simulink model "V1"  (Simulink 8.9)
settings: Solver=VariableStepAuto  StartTime=0.0  StopTime=5  RelTol=1e-3
values from neighbouring files (symbols this model uses):
  Fz = m*g/2    (= 3924)    [variabeln.m]    (also in variabeln_v2.m)
  J = 1    [variabeln.m]    (also in variabeln_v2.m)
  m = 800    [variabeln.m]    (also in variabeln_v2.m)
  r = 0.25    [variabeln.m]    (also in variabeln_v2.m)
  theta1 = 1.28    [variabeln.m]    (also in variabeln_v2.m)
  theta2 = 23.99    [variabeln.m]    (also in variabeln_v2.m)
  theta3 = 0.52    [variabeln.m]    (also in variabeln_v2.m)
  v0 = 10    [variabeln.m]    (also in variabeln_v2.m = 50)
settings Model: Creator=frede  LastModifiedBy=frede
settings DataIOCC: LimitDataPoints=off  SaveFormat=Dataset  SignalLoggingSaveFormat=Dataset
settings OptimizationCC: LifeSpan=auto
settings DebuggingCC: UnderspecifiedInitializationDetection=Simplified  MergeDetectMultiDrivingBlocksExec=error  FcnCallInpInsideContextMsg=error  StateNameClashWarn=none  SFUnexpectedBacktrackingDiag=error  SFNoUnconditionalDefaultTransitionDiag=error  SFExecutionAtInitializationDiag=warning
settings HardwareCC: ProdBitPerPointer=64  ProdBitPerSizeT=64  ProdBitPerPtrDiffT=64  ProdLargestAtomicFloat=Float  ProdIntDivRoundTo=Zero  ProdEndianess=LittleEndian  ProdWordSize=64  ProdHWDeviceType=Intel->x86-64 (Windows64)
settings ModelReferenceCC: PropagateSignalLabelsOutOfModel=on
settings GRTTargetCC: TargetLangStandard=C99 (ISO)  GeneratePreprocessorConditionals=Use local settings  CombineOutputUpdateFcns=on  GRTInterface=off
settings ConfigComp: CovMetricSettings=dwe  CovHtmlReporting=off  CovSaveCumulativeToWorkspaceVar=off  CovSaveSingleToWorkspaceVar=off  CovExternalEMLEnable=on

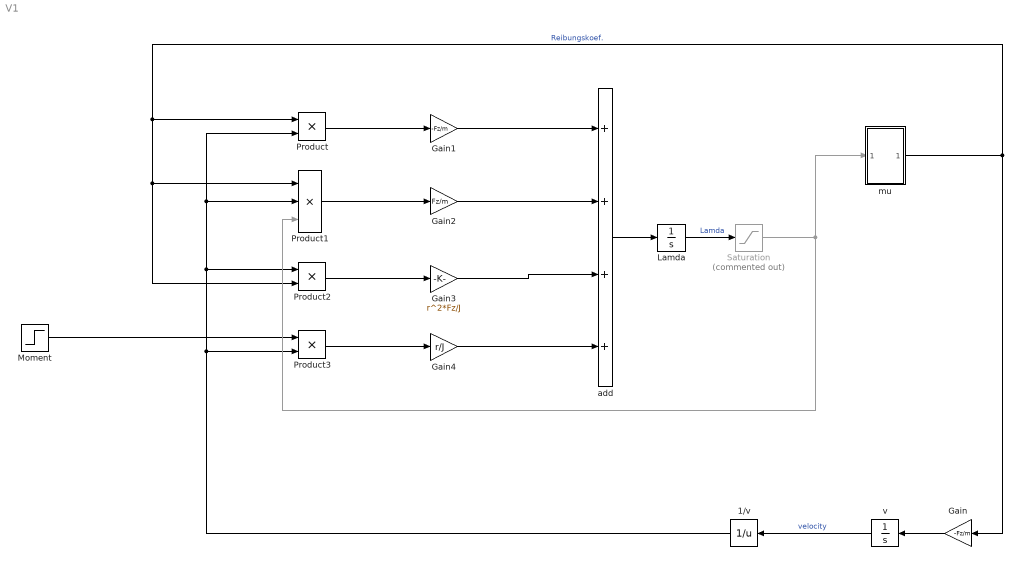
== system V1 ==
  "1/v " : Math  Operator=reciprocal  SaturateOnIntegerOverflow=on
  Gain : Gain  Gain=-Fz/m
  Gain1 : Gain  Gain=-Fz/m
  Gain2 : Gain  Gain=Fz/m
  Gain3 : Gain  Gain=r^2*Fz/J
  Gain4 : Gain  Gain=r/J
  Lamda : Integrator  IgnoreLimit=on
  Moment : Step  After=10  SampleTime=0
  Product : Product
  Product1 : Product  Inputs=3
  Product2 : Product
  Product3 : Product
  Saturation : Saturate  Commented=on  UpperLimit=1
  add : Sum  Inputs=++++
  mu : Subsystem
  v : Integrator  InitialCondition=v0
  wires:
  mu/1(Out1) -> Product2/2, Product1/1, Product/1, Gain/1  "Reibungskoef."
  Gain/1 -> v/1
  "1/v "/1 -> Product3/2, Product2/1, Product1/2, Product/2
  Product/1 -> Gain1/1
  Gain1/1 -> add/1
  add/1 -> Lamda/1
  Product1/1 -> Gain2/1
  Gain2/1 -> add/2
  Product2/1 -> Gain3/1
  Gain3/1 -> add/3
  Gain4/1 -> add/4
  Product3/1 -> Gain4/1
  Moment/1 -> Product3/1
  v/1 -> "1/v "/1  "velocity"
  Lamda/1 -> Saturation/1  "Lamda"
  Saturation/1 -> Product1/3, mu/1(In1)

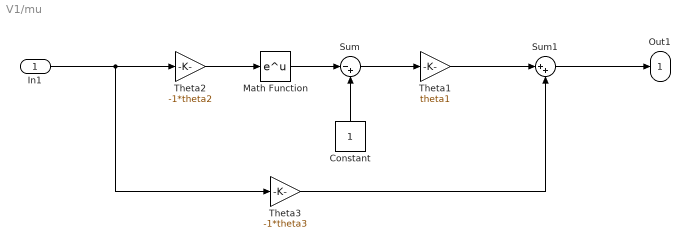
== system V1/mu ==
  In1 : Inport
  Constant : Constant
  Math Function : Math  SaturateOnIntegerOverflow=on
  Sum : Sum  Inputs=|-+
  Sum1 : Sum  Inputs=|++
  Theta1 : Gain  Gain=theta1
  "Theta2 " : Gain  Gain=-1*theta2
  "Theta3 " : Gain  Gain=-1*theta3
  Out1 : Outport
  wires:
  In1/1 -> "Theta3 "/1, "Theta2 "/1
  Math Function/1 -> Sum/1
  Sum/1 -> Theta1/1
  "Theta3 "/1 -> Sum1/2
  Theta1/1 -> Sum1/1
  Sum1/1 -> Out1/1
  "Theta2 "/1 -> Math Function/1
  Constant/1 -> Sum/2
